simulink model "LR3_BakVoda"  (R2015b)
settings: Solver=VariableStepAuto  StartTime=0.0  StopTime=100.0  RelTol=1e-3
values from neighbouring files (symbols this model uses):
  fisREG = readfis('stage3gauss')    [LR_3_BakVoda.m]
  Ki = 0.1    [LR_3_BakVoda.m]
  Kz = 1.2    [LR_3_BakVoda.m]
  Sb = 8.0    (= 8)    [LR_3_BakVoda.m]
undefined symbols (not defined in the file or in its folder): sigbuilder_block
libraries: fuzblock x1
settings Model: Creator=Сергей  LastModifiedBy=сериков

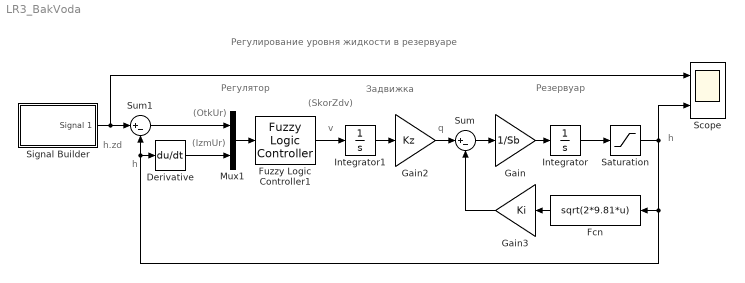
== system LR3_BakVoda ==
  note: h.zd
  note: Резервуар
  note: Регулирование уровня жидкости в резервуаре
  note: Регулятор
  note: Задвижка
  note: h
  note: v
  note: h
  note: q
  note: (SkorZdv)
  note: (OtkUr)
  note: (IzmUr)
  Derivative : Derivative
  Fcn : Fcn  Expr=sqrt(2*9.81*u)
  Fuzzy Logic Controller1 : fuzblock/Fuzzy Logic  Controller  fis=[fisREG]
  Gain : Gain  Gain=1/Sb
  Gain2 : Gain  Gain=Kz
  Gain3 : Gain  Gain=Ki
  Integrator : Integrator
  Integrator1 : Integrator
  Mux1 : Mux  Inputs=2
  Saturation : Saturate  UpperLimit=100  LowerLimit=0
  Scope : Scope  NumInputPorts=2
  Signal Builder : Subsystem  Tag=STV Subsys  LoadFcn=sigbuilder_block('load');  StartFcn=sigbuilder_block('start');  StopFcn=sigbuilder_block('stop');  ClipboardFcn=sigbuilder_block('clipboard');  mask(Sigbuilder block){}
      mask help: Simulink:masks:SigbuilderBlock_MD
      mask init:
      | if ~strcmp(get_param(bdroot(gcbh),'SimulationStatus'),'stopped') tuvar = sigbuilder_block('maskInit'); end
      settings: CopyFcn=sigbuilder_block('copy');  DeleteFcn=sigbuilder_block('delete');  ModelCloseFcn=sigbuilder_block('modelClose');  PreSaveFcn=sigbuilder_block('preSave');  PauseFcn=sigbuilder_block('pause');  ContinueFcn=sigbuilder_block('continue');  NameChangeFcn=sigbuilder_block('namechange');  OpenFcn=sigbuilder_block('open',[63.75 114.75 550.5 399.75 ]);  CloseFcn=sigbuilder_block('close');
      mask Display: plot(0, 0, 100, 100,[2, 2, 32, 32, 2], [68, 8, 8, 68, 68],[32, 2], [38, 38], [32, 19, 2],[53, 60, 44], [32, 17, 17, 2],[16, 16, 31, 31]);txt = getActiveGroup(gcbh);text(2, 100, txt,'verticalAlignment', 'top');
  Sum : Sum  Inputs=|+-
  Sum1 : Sum  Inputs=|+-
  wires:
  Gain/1 -> Integrator/1
  Sum/1 -> Gain/1
  Fcn/1 -> Gain3/1
  Gain3/1 -> Sum/2
  Signal Builder/1(Signal 1) -> Scope/1, Sum1/1
  Mux1/1 -> Fuzzy Logic Controller1/1
  Sum1/1 -> Mux1/1
  Derivative/1 -> Mux1/2
  Integrator/1 -> Saturation/1
  Saturation/1 -> Scope/2, Fcn/1, Derivative/1, Sum1/2
  Gain2/1 -> Sum/1
  Integrator1/1 -> Gain2/1
  Fuzzy Logic Controller1/1 -> Integrator1/1

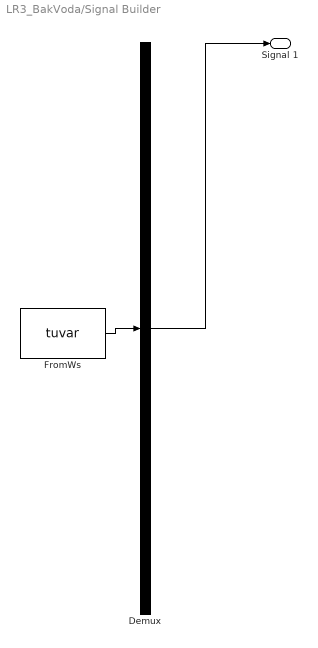
== system LR3_BakVoda/Signal Builder ==
  Demux : Demux  Tag=STV Demux  Outputs=1
  FromWs : FromWorkspace  Tag=STV FromWs  VariableName=tuvar  SampleTime=0
      SigBuilderData=|
      | common.afterFinalStr = 'Extrapolate'
      | common.sampleTime = 0
      | dataSet.timeRange = [0 100]
      | dataSet.name = 'Group 1'
      | sbobj.Groups.Name = 'Group 1'
      | sbobj.Groups.Signals.Name = 'Signal 1'
      | sbobj.Groups.Signals.XData = [0 1 1 60 60 100]
      | sbobj.Groups.Signals.YData = [0 0 1 1 0.4 0.395]
      | sbobj.Groups.TimeRange = [0 100]
  Signal 1 : Outport  Tag=STV Outport
  wires:
  Demux/1 -> Signal 1/1
  FromWs/1 -> Demux/1
